simulink library "time2Rotations"  (R2018b)
settings: Solver=VariableStepAuto  StartTime=0.0  StopTime=10.0  RelTol=1e-3
libraries: rotations_Lib x1, time_lib x1
settings Model: Creator=IvanMachuca  LastModifiedBy=devantormey

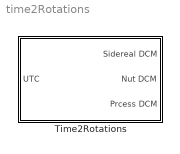
== system time2Rotations ==
  "Time2Rotations " : Subsystem

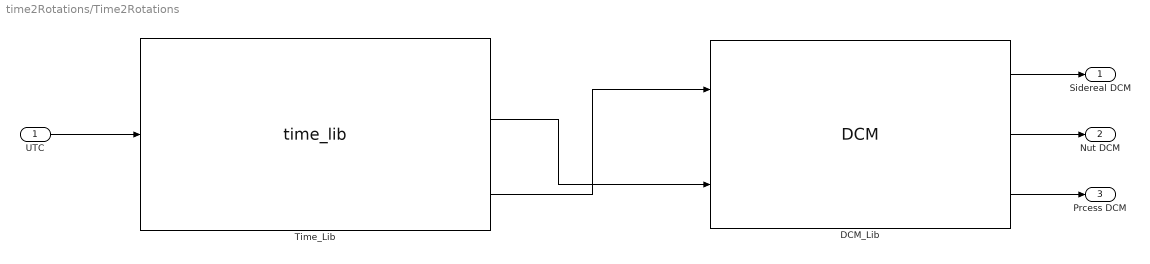
== system time2Rotations/Time2Rotations  ==
  UTC : Inport
  "DCM_Lib " : rotations_Lib/DCM   SystemSampleTime=-1
  "Time_Lib " : time_lib/time_lib    SystemSampleTime=-1
  Sidereal DCM : Outport
  "Nut DCM " : Outport  Port=2
  "Prcess DCM " : Outport  Port=3
  wires:
  "Time_Lib "/6 -> "DCM_Lib "/2
  "Time_Lib "/11 -> "DCM_Lib "/1
  UTC/1 -> "Time_Lib "/1
  "DCM_Lib "/1 -> Sidereal DCM/1
  "DCM_Lib "/2 -> "Nut DCM "/1
  "DCM_Lib "/3 -> "Prcess DCM "/1
